simulink model "traffic"  (R2016a)
settings: Solver=FixedStepDiscrete  StartTime=0.0  StopTime=inf  FixedStep=0.1  RelTol=1e-3
libraries: arduinolib x3
settings Model: ExtModeTrigDuration=2  Creator=areej_ofamech  LastModifiedBy=areej_ofamech
settings SolverCC: AutoInsertRateTranBlk=on
settings DataIOCC: LimitDataPoints=on
settings OptimizationCC: OptimizeModelRefInitCode=on  LifeSpan=Inf  MaxStackSize=64
settings DebuggingCC: AllowSymbolicDim=off
settings HardwareCC: ProdBitPerInt=16  ProdBitPerPointer=16  ProdLargestAtomicFloat=None  ProdWordSize=8  ProdHWDeviceType=Atmel->AVR
settings RTWCC: SystemTargetFile=ert.tlc  HardwareBoard=Arduino Uno  TemplateMakefile=ert_default_tmf  GenerateReport=on  Toolchain=Arduino AVR v1.6.1  BuildConfiguration=Faster Runs  IncludeHyperlinkInReport=on  LaunchReport=on  GenerateTraceInfo=on  GenerateTraceReport=on  GenerateTraceReportSl=on  GenerateTraceReportSf=on  GenerateTraceReportEml=on
settings CodeAppCC: ForceParamTrailComments=on  IgnoreCustomStorageClasses=off  OperatorAnnotations=on  SimulinkDataObjDesc=on  SFDataObjDesc=on  MATLABFcnDesc=on  InsertBlockDesc=on  MATLABSourceComments=on
settings ERTTargetCC: SupportContinuousTime=on  SupportVariableSizeSignals=on
settings ConfigComp: CovModelRefEnable=Off  CovSFcnEnable=off

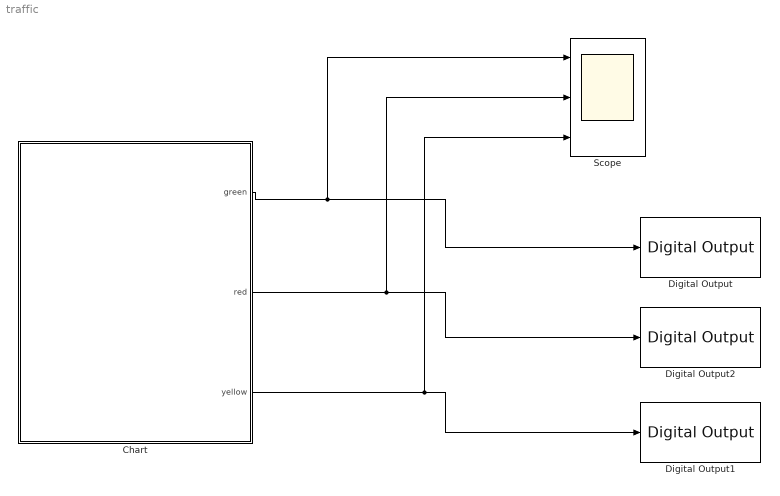
== system traffic ==
  Chart : Stateflow chart  TreatAsAtomicUnit=on
  Digital Output : arduinolib/Digital Output  pinNumber=9  blockPlatform=arduino
  Digital Output1 : arduinolib/Digital Output  pinNumber=7  blockPlatform=arduino
  Digital Output2 : arduinolib/Digital Output  pinNumber=8  blockPlatform=arduino
  Scope : Scope  NumInputPorts=3
  wires:
  Chart/1(green) -> Scope/1, Digital Output/1
  Chart/2(red) -> Scope/2, Digital Output2/1
  Chart/3(yellow) -> Scope/3, Digital Output1/1

== stateflow chart traffic/Chart ==
  state Init
    state init
      entry: ctr =0;
    state transition
      entry: red=0;
      yellow =0;
      green =0;
    state init_blink
      entry: red=1;
      yellow =1;
      green =1;
      ctr =ctr+1;
    (default) -> init
    transition -> init_blink : [after(5,sec)&&ctr~=3]
    init -> init_blink
    init_blink -> transition : [after(5,sec)]
  state Traffic
    state Red
      entry: red =1;
    state Green
      entry: green =1;
    state Yellow
      entry: yellow = 1;
    Green -> Red : [after(5,sec)]{green=0 ;after(5,sec);}
    (default) -> Red
    Red -> Yellow : [after(5,sec)]{red=0 ;after(5,sec);}
    Yellow -> Green : [after(5,sec)]{yellow=0 ;after(5,sec);}
  (default) -> Init
  Init -> Traffic : [after(5,sec)&&ctr==3]
  data: green output; red output; yellow output; ctr local
